simulink model "thermostat"  (R2014b)
settings: Solver=ode1  StartTime=0.0  StopTime=100  FixedStep=0.0001  MaxStep=0.0001  RelTol=1e-3
(part 1 of 2)
settings Model: Creator=sand080  LastModifiedBy=nall426
settings DataIOCC: LimitDataPoints=off
settings RTWCC: CustomInitializer=gettimeofday(&t0, 0);
settings RTWCC: CustomSourceCode=|
  | int gettimeofday(struct timeval * tp, struct timezone * tzp)
  | {
  |     // Note: some broken versions only have 8 trailing zero's, the correct epoch has 9 trailing zero's
  |     static const uint64_t EPOCH = ((uint64_t) 116444736000000000ULL);
  | 
  |     SYSTEMTIME  system_time;
  |     FILETIME    file_time;
  |     uint64_t    time;
  | 
  | 	GetSystemTime( &system_time );
  |     SystemTimeToFileTime( &system_time, &file_time );
  |     time =  ((uint64_t)file_time.dwLowDateTime )      ;
  |     time += ((uint64_t)file_time.dwHighDateTime) << 32;
  | 
  |     tp->tv_sec  = (long) ((time - EPOCH) / 10000000L);
  |     tp->tv_usec = (long) (system_time.wMilliseconds * 1000);
  |     return 0;
  | }
  | 
  | struct timeval t0, t1;
settings RTWCC: CustomHeaderCode=|
  | #include <stdint.h> // portable: uint64_t   MSVC: __int64
  | #include <Windows.h>
settings RTWCC: CustomTerminator=|
  | gettimeofday(&t1, 0);
  | 
  | long elapsed = (t1.tv_sec-t0.tv_sec)*1000000 + t1.tv_usec-t0.tv_usec;
  | printf("Time taken: %ld microseconds (%.3f seconds)\n", elapsed, (elapsed / 1000000.0));

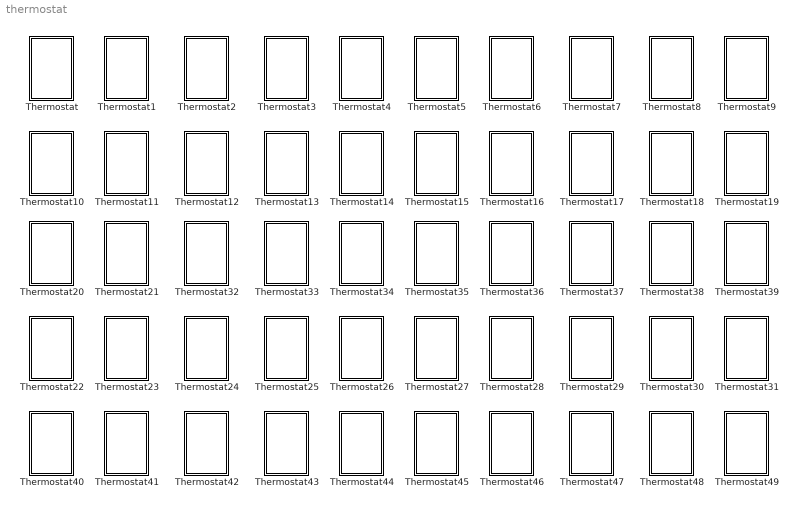
== system thermostat ==
  Thermostat : Subsystem
  Thermostat1 : Subsystem
  Thermostat10 : Subsystem
  Thermostat11 : Subsystem
  Thermostat12 : Subsystem
  Thermostat13 : Subsystem
  Thermostat14 : Subsystem
  Thermostat15 : Subsystem
  Thermostat16 : Subsystem
  Thermostat17 : Subsystem
  Thermostat18 : Subsystem
  Thermostat19 : Subsystem
  Thermostat2 : Subsystem
  Thermostat20 : Subsystem
  Thermostat21 : Subsystem
  Thermostat22 : Subsystem
  Thermostat23 : Subsystem
  Thermostat24 : Subsystem
  Thermostat25 : Subsystem
  Thermostat26 : Subsystem
  Thermostat27 : Subsystem
  Thermostat28 : Subsystem
  Thermostat29 : Subsystem
  Thermostat3 : Subsystem
  Thermostat30 : Subsystem
  Thermostat31 : Subsystem
  Thermostat32 : Subsystem
  Thermostat33 : Subsystem
  Thermostat34 : Subsystem
  Thermostat35 : Subsystem
  Thermostat36 : Subsystem
  Thermostat37 : Subsystem
  Thermostat38 : Subsystem
  Thermostat39 : Subsystem
  Thermostat4 : Subsystem
  Thermostat40 : Subsystem
  Thermostat41 : Subsystem
  Thermostat42 : Subsystem
  Thermostat43 : Subsystem
  Thermostat44 : Subsystem
  Thermostat45 : Subsystem
  Thermostat46 : Subsystem
  Thermostat47 : Subsystem
  Thermostat48 : Subsystem
  Thermostat49 : Subsystem
  Thermostat5 : Subsystem
  Thermostat6 : Subsystem
  Thermostat7 : Subsystem
  Thermostat8 : Subsystem
  Thermostat9 : Subsystem

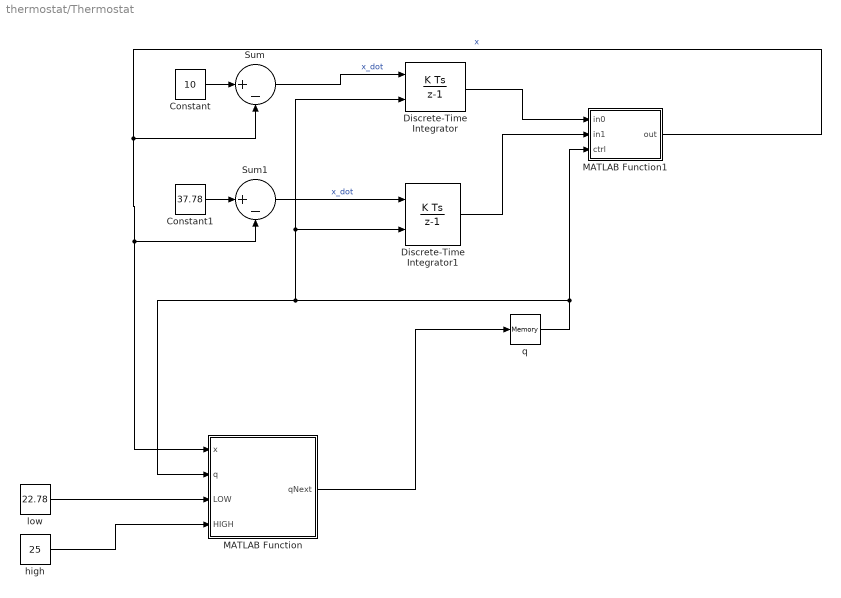
== system thermostat/Thermostat ==
  Constant : Constant  Value=10
  Constant1 : Constant  Value=37.78
  Discrete-Time Integrator : DiscreteIntegrator  ExternalReset=either  InitialCondition=25  InitialConditionSetting=State (most efficient)  SampleTime=-1
  Discrete-Time Integrator1 : DiscreteIntegrator  ExternalReset=either  InitialCondition=22.78  InitialConditionSetting=State (most efficient)  SampleTime=-1
  MATLAB Function : MATLAB Function  TreatAsAtomicUnit=on
  MATLAB Function1 : MATLAB Function  TreatAsAtomicUnit=on
  Sum : Sum  Inputs=|+-
  Sum1 : Sum  Inputs=|+-
  high : Constant  Value=25
  low : Constant  Value=22.78
  q : Memory
  wires:
  MATLAB Function/1(qNext) -> q/1
  Constant/1 -> Sum/1
  Sum/1 -> Discrete-Time Integrator/1  "x_dot"
  Discrete-Time Integrator1/1 -> MATLAB Function1/2(in1)
  Constant1/1 -> Sum1/1
  Sum1/1 -> Discrete-Time Integrator1/1  "x_dot"
  Discrete-Time Integrator/1 -> MATLAB Function1/1(in0)
  MATLAB Function1/1(out) -> Sum/2, MATLAB Function/1(x), Sum1/2  "x"
  low/1 -> MATLAB Function/3(LOW)
  high/1 -> MATLAB Function/4(HIGH)
  q/1 -> MATLAB Function1/3(ctrl), Discrete-Time Integrator1/2, Discrete-Time Integrator/2, MATLAB Function/2(q)

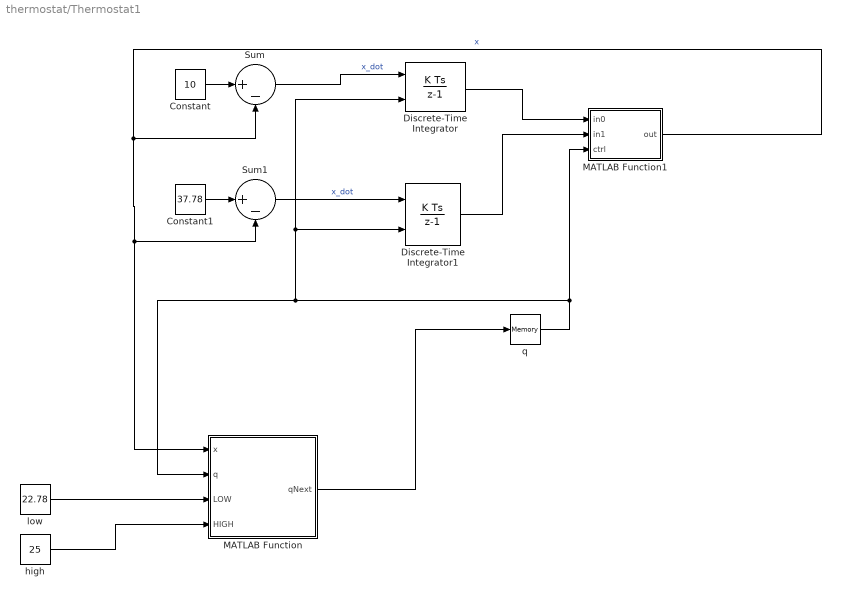
== system thermostat/Thermostat1 ==
  Constant : Constant  Value=10
  Constant1 : Constant  Value=37.78
  Discrete-Time Integrator : DiscreteIntegrator  ExternalReset=either  InitialCondition=25  InitialConditionSetting=State (most efficient)  SampleTime=-1
  Discrete-Time Integrator1 : DiscreteIntegrator  ExternalReset=either  InitialCondition=22.78  InitialConditionSetting=State (most efficient)  SampleTime=-1
  MATLAB Function : MATLAB Function  TreatAsAtomicUnit=on
  MATLAB Function1 : MATLAB Function  TreatAsAtomicUnit=on
  Sum : Sum  Inputs=|+-
  Sum1 : Sum  Inputs=|+-
  high : Constant  Value=25
  low : Constant  Value=22.78
  q : Memory
  wires:
  MATLAB Function/1(qNext) -> q/1
  Constant/1 -> Sum/1
  Sum/1 -> Discrete-Time Integrator/1  "x_dot"
  Discrete-Time Integrator1/1 -> MATLAB Function1/2(in1)
  Constant1/1 -> Sum1/1
  Sum1/1 -> Discrete-Time Integrator1/1  "x_dot"
  Discrete-Time Integrator/1 -> MATLAB Function1/1(in0)
  MATLAB Function1/1(out) -> Sum/2, MATLAB Function/1(x), Sum1/2  "x"
  low/1 -> MATLAB Function/3(LOW)
  high/1 -> MATLAB Function/4(HIGH)
  q/1 -> MATLAB Function1/3(ctrl), Discrete-Time Integrator1/2, Discrete-Time Integrator/2, MATLAB Function/2(q)

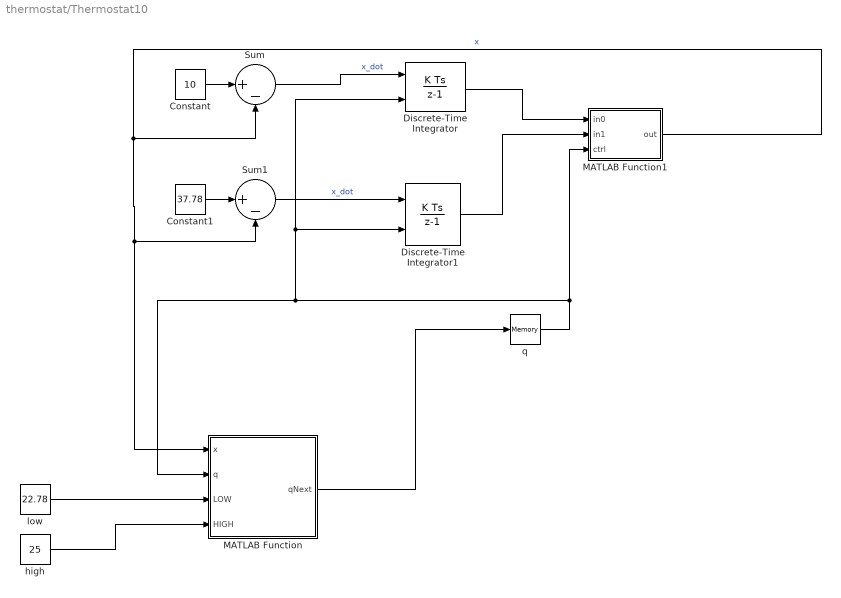
== system thermostat/Thermostat10 ==
  Constant : Constant  Value=10
  Constant1 : Constant  Value=37.78
  Discrete-Time Integrator : DiscreteIntegrator  ExternalReset=either  InitialCondition=25  InitialConditionSetting=State (most efficient)  SampleTime=-1
  Discrete-Time Integrator1 : DiscreteIntegrator  ExternalReset=either  InitialCondition=22.78  InitialConditionSetting=State (most efficient)  SampleTime=-1
  MATLAB Function : MATLAB Function  TreatAsAtomicUnit=on
  MATLAB Function1 : MATLAB Function  TreatAsAtomicUnit=on
  Sum : Sum  Inputs=|+-
  Sum1 : Sum  Inputs=|+-
  high : Constant  Value=25
  low : Constant  Value=22.78
  q : Memory
  wires:
  MATLAB Function/1(qNext) -> q/1
  Constant/1 -> Sum/1
  Sum/1 -> Discrete-Time Integrator/1  "x_dot"
  Discrete-Time Integrator1/1 -> MATLAB Function1/2(in1)
  Constant1/1 -> Sum1/1
  Sum1/1 -> Discrete-Time Integrator1/1  "x_dot"
  Discrete-Time Integrator/1 -> MATLAB Function1/1(in0)
  MATLAB Function1/1(out) -> Sum/2, MATLAB Function/1(x), Sum1/2  "x"
  low/1 -> MATLAB Function/3(LOW)
  high/1 -> MATLAB Function/4(HIGH)
  q/1 -> MATLAB Function1/3(ctrl), Discrete-Time Integrator1/2, Discrete-Time Integrator/2, MATLAB Function/2(q)

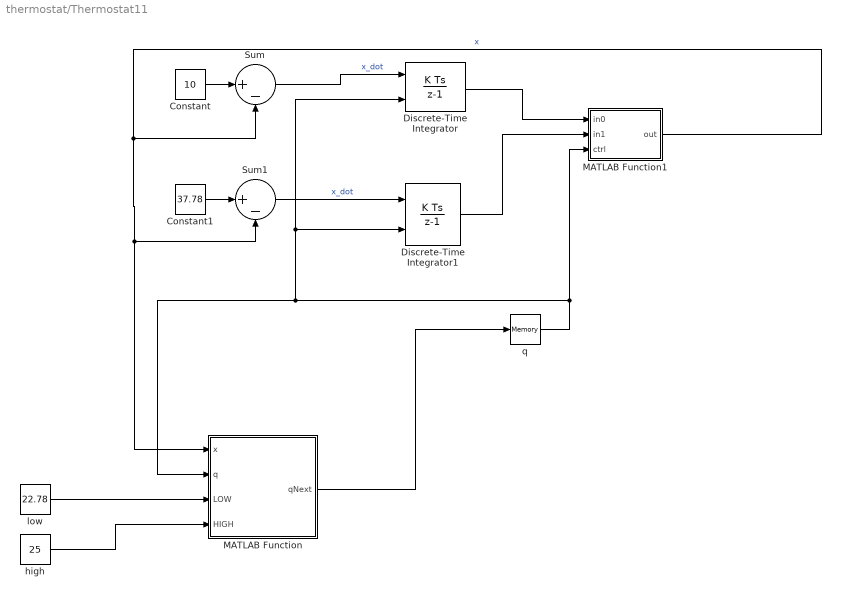
== system thermostat/Thermostat11 ==
  Constant : Constant  Value=10
  Constant1 : Constant  Value=37.78
  Discrete-Time Integrator : DiscreteIntegrator  ExternalReset=either  InitialCondition=25  InitialConditionSetting=State (most efficient)  SampleTime=-1
  Discrete-Time Integrator1 : DiscreteIntegrator  ExternalReset=either  InitialCondition=22.78  InitialConditionSetting=State (most efficient)  SampleTime=-1
  MATLAB Function : MATLAB Function  TreatAsAtomicUnit=on
  MATLAB Function1 : MATLAB Function  TreatAsAtomicUnit=on
  Sum : Sum  Inputs=|+-
  Sum1 : Sum  Inputs=|+-
  high : Constant  Value=25
  low : Constant  Value=22.78
  q : Memory
  wires:
  MATLAB Function/1(qNext) -> q/1
  Constant/1 -> Sum/1
  Sum/1 -> Discrete-Time Integrator/1  "x_dot"
  Discrete-Time Integrator1/1 -> MATLAB Function1/2(in1)
  Constant1/1 -> Sum1/1
  Sum1/1 -> Discrete-Time Integrator1/1  "x_dot"
  Discrete-Time Integrator/1 -> MATLAB Function1/1(in0)
  MATLAB Function1/1(out) -> Sum/2, MATLAB Function/1(x), Sum1/2  "x"
  low/1 -> MATLAB Function/3(LOW)
  high/1 -> MATLAB Function/4(HIGH)
  q/1 -> MATLAB Function1/3(ctrl), Discrete-Time Integrator1/2, Discrete-Time Integrator/2, MATLAB Function/2(q)

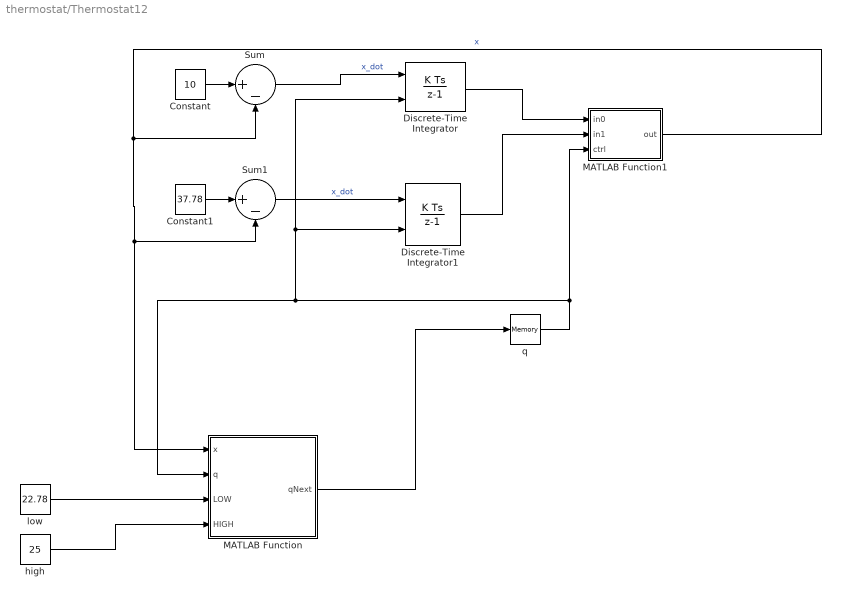
== system thermostat/Thermostat12 ==
  Constant : Constant  Value=10
  Constant1 : Constant  Value=37.78
  Discrete-Time Integrator : DiscreteIntegrator  ExternalReset=either  InitialCondition=25  InitialConditionSetting=State (most efficient)  SampleTime=-1
  Discrete-Time Integrator1 : DiscreteIntegrator  ExternalReset=either  InitialCondition=22.78  InitialConditionSetting=State (most efficient)  SampleTime=-1
  MATLAB Function : MATLAB Function  TreatAsAtomicUnit=on
  MATLAB Function1 : MATLAB Function  TreatAsAtomicUnit=on
  Sum : Sum  Inputs=|+-
  Sum1 : Sum  Inputs=|+-
  high : Constant  Value=25
  low : Constant  Value=22.78
  q : Memory
  wires:
  MATLAB Function/1(qNext) -> q/1
  Constant/1 -> Sum/1
  Sum/1 -> Discrete-Time Integrator/1  "x_dot"
  Discrete-Time Integrator1/1 -> MATLAB Function1/2(in1)
  Constant1/1 -> Sum1/1
  Sum1/1 -> Discrete-Time Integrator1/1  "x_dot"
  Discrete-Time Integrator/1 -> MATLAB Function1/1(in0)
  MATLAB Function1/1(out) -> Sum/2, MATLAB Function/1(x), Sum1/2  "x"
  low/1 -> MATLAB Function/3(LOW)
  high/1 -> MATLAB Function/4(HIGH)
  q/1 -> MATLAB Function1/3(ctrl), Discrete-Time Integrator1/2, Discrete-Time Integrator/2, MATLAB Function/2(q)

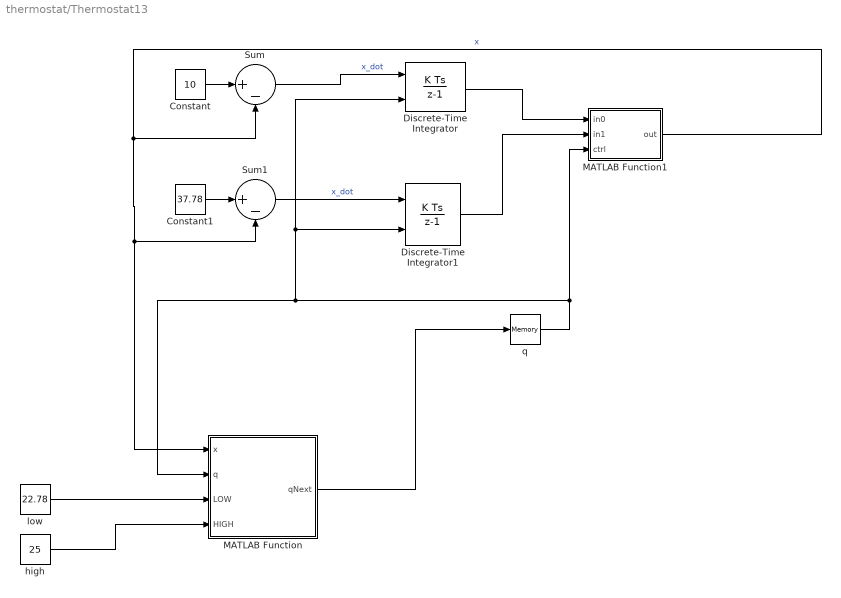
== system thermostat/Thermostat13 ==
  Constant : Constant  Value=10
  Constant1 : Constant  Value=37.78
  Discrete-Time Integrator : DiscreteIntegrator  ExternalReset=either  InitialCondition=25  InitialConditionSetting=State (most efficient)  SampleTime=-1
  Discrete-Time Integrator1 : DiscreteIntegrator  ExternalReset=either  InitialCondition=22.78  InitialConditionSetting=State (most efficient)  SampleTime=-1
  MATLAB Function : MATLAB Function  TreatAsAtomicUnit=on
  MATLAB Function1 : MATLAB Function  TreatAsAtomicUnit=on
  Sum : Sum  Inputs=|+-
  Sum1 : Sum  Inputs=|+-
  high : Constant  Value=25
  low : Constant  Value=22.78
  q : Memory
  wires:
  MATLAB Function/1(qNext) -> q/1
  Constant/1 -> Sum/1
  Sum/1 -> Discrete-Time Integrator/1  "x_dot"
  Discrete-Time Integrator1/1 -> MATLAB Function1/2(in1)
  Constant1/1 -> Sum1/1
  Sum1/1 -> Discrete-Time Integrator1/1  "x_dot"
  Discrete-Time Integrator/1 -> MATLAB Function1/1(in0)
  MATLAB Function1/1(out) -> Sum/2, MATLAB Function/1(x), Sum1/2  "x"
  low/1 -> MATLAB Function/3(LOW)
  high/1 -> MATLAB Function/4(HIGH)
  q/1 -> MATLAB Function1/3(ctrl), Discrete-Time Integrator1/2, Discrete-Time Integrator/2, MATLAB Function/2(q)

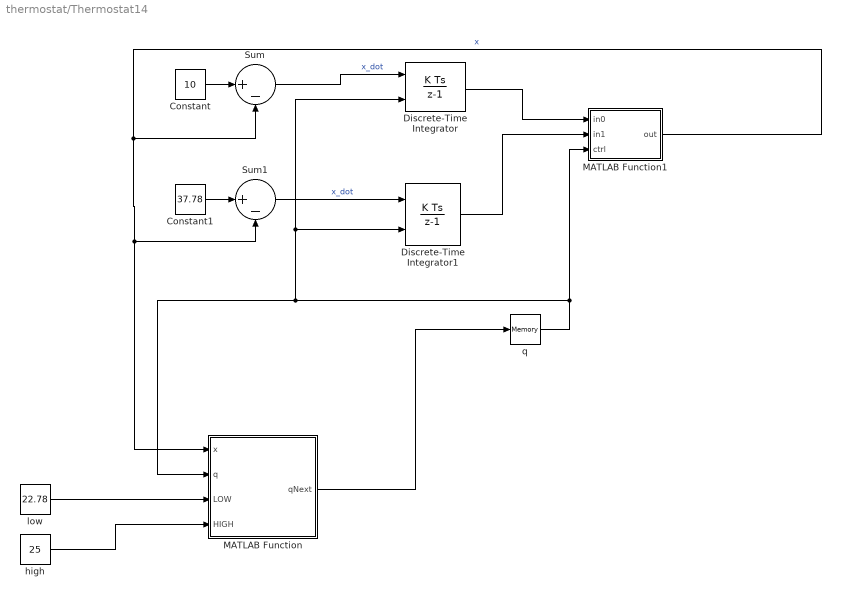
== system thermostat/Thermostat14 ==
  Constant : Constant  Value=10
  Constant1 : Constant  Value=37.78
  Discrete-Time Integrator : DiscreteIntegrator  ExternalReset=either  InitialCondition=25  InitialConditionSetting=State (most efficient)  SampleTime=-1
  Discrete-Time Integrator1 : DiscreteIntegrator  ExternalReset=either  InitialCondition=22.78  InitialConditionSetting=State (most efficient)  SampleTime=-1
  MATLAB Function : MATLAB Function  TreatAsAtomicUnit=on
  MATLAB Function1 : MATLAB Function  TreatAsAtomicUnit=on
  Sum : Sum  Inputs=|+-
  Sum1 : Sum  Inputs=|+-
  high : Constant  Value=25
  low : Constant  Value=22.78
  q : Memory
  wires:
  MATLAB Function/1(qNext) -> q/1
  Constant/1 -> Sum/1
  Sum/1 -> Discrete-Time Integrator/1  "x_dot"
  Discrete-Time Integrator1/1 -> MATLAB Function1/2(in1)
  Constant1/1 -> Sum1/1
  Sum1/1 -> Discrete-Time Integrator1/1  "x_dot"
  Discrete-Time Integrator/1 -> MATLAB Function1/1(in0)
  MATLAB Function1/1(out) -> Sum/2, MATLAB Function/1(x), Sum1/2  "x"
  low/1 -> MATLAB Function/3(LOW)
  high/1 -> MATLAB Function/4(HIGH)
  q/1 -> MATLAB Function1/3(ctrl), Discrete-Time Integrator1/2, Discrete-Time Integrator/2, MATLAB Function/2(q)

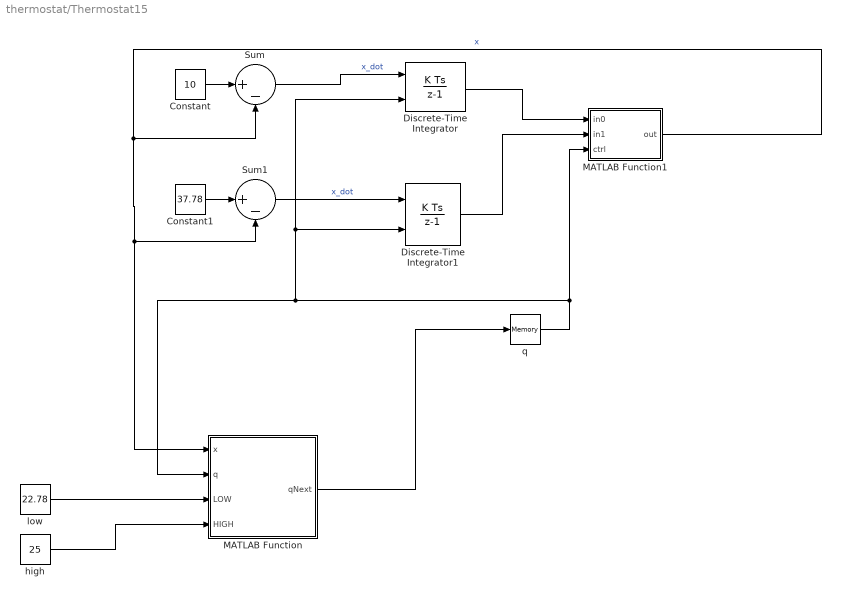
== system thermostat/Thermostat15 ==
  Constant : Constant  Value=10
  Constant1 : Constant  Value=37.78
  Discrete-Time Integrator : DiscreteIntegrator  ExternalReset=either  InitialCondition=25  InitialConditionSetting=State (most efficient)  SampleTime=-1
  Discrete-Time Integrator1 : DiscreteIntegrator  ExternalReset=either  InitialCondition=22.78  InitialConditionSetting=State (most efficient)  SampleTime=-1
  MATLAB Function : MATLAB Function  TreatAsAtomicUnit=on
  MATLAB Function1 : MATLAB Function  TreatAsAtomicUnit=on
  Sum : Sum  Inputs=|+-
  Sum1 : Sum  Inputs=|+-
  high : Constant  Value=25
  low : Constant  Value=22.78
  q : Memory
  wires:
  MATLAB Function/1(qNext) -> q/1
  Constant/1 -> Sum/1
  Sum/1 -> Discrete-Time Integrator/1  "x_dot"
  Discrete-Time Integrator1/1 -> MATLAB Function1/2(in1)
  Constant1/1 -> Sum1/1
  Sum1/1 -> Discrete-Time Integrator1/1  "x_dot"
  Discrete-Time Integrator/1 -> MATLAB Function1/1(in0)
  MATLAB Function1/1(out) -> Sum/2, MATLAB Function/1(x), Sum1/2  "x"
  low/1 -> MATLAB Function/3(LOW)
  high/1 -> MATLAB Function/4(HIGH)
  q/1 -> MATLAB Function1/3(ctrl), Discrete-Time Integrator1/2, Discrete-Time Integrator/2, MATLAB Function/2(q)

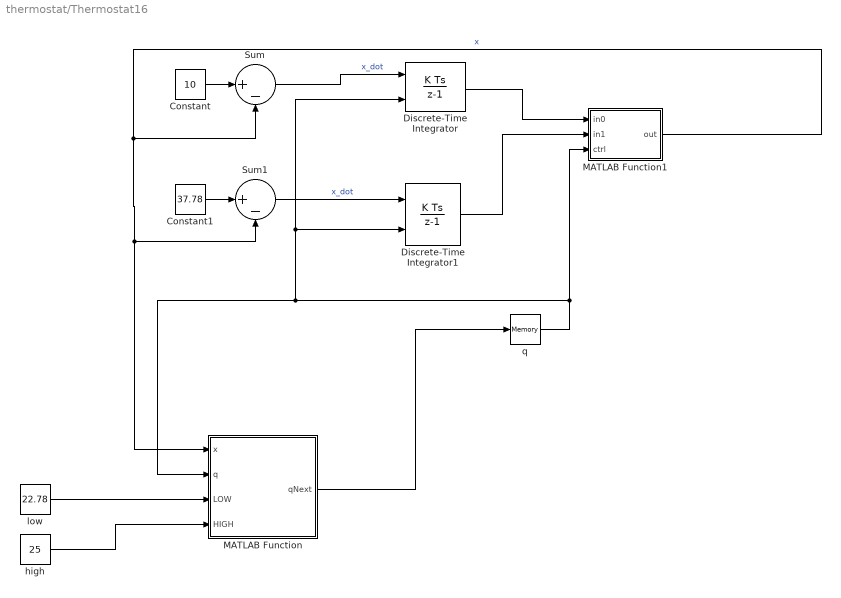
== system thermostat/Thermostat16 ==
  Constant : Constant  Value=10
  Constant1 : Constant  Value=37.78
  Discrete-Time Integrator : DiscreteIntegrator  ExternalReset=either  InitialCondition=25  InitialConditionSetting=State (most efficient)  SampleTime=-1
  Discrete-Time Integrator1 : DiscreteIntegrator  ExternalReset=either  InitialCondition=22.78  InitialConditionSetting=State (most efficient)  SampleTime=-1
  MATLAB Function : MATLAB Function  TreatAsAtomicUnit=on
  MATLAB Function1 : MATLAB Function  TreatAsAtomicUnit=on
  Sum : Sum  Inputs=|+-
  Sum1 : Sum  Inputs=|+-
  high : Constant  Value=25
  low : Constant  Value=22.78
  q : Memory
  wires:
  MATLAB Function/1(qNext) -> q/1
  Constant/1 -> Sum/1
  Sum/1 -> Discrete-Time Integrator/1  "x_dot"
  Discrete-Time Integrator1/1 -> MATLAB Function1/2(in1)
  Constant1/1 -> Sum1/1
  Sum1/1 -> Discrete-Time Integrator1/1  "x_dot"
  Discrete-Time Integrator/1 -> MATLAB Function1/1(in0)
  MATLAB Function1/1(out) -> Sum/2, MATLAB Function/1(x), Sum1/2  "x"
  low/1 -> MATLAB Function/3(LOW)
  high/1 -> MATLAB Function/4(HIGH)
  q/1 -> MATLAB Function1/3(ctrl), Discrete-Time Integrator1/2, Discrete-Time Integrator/2, MATLAB Function/2(q)

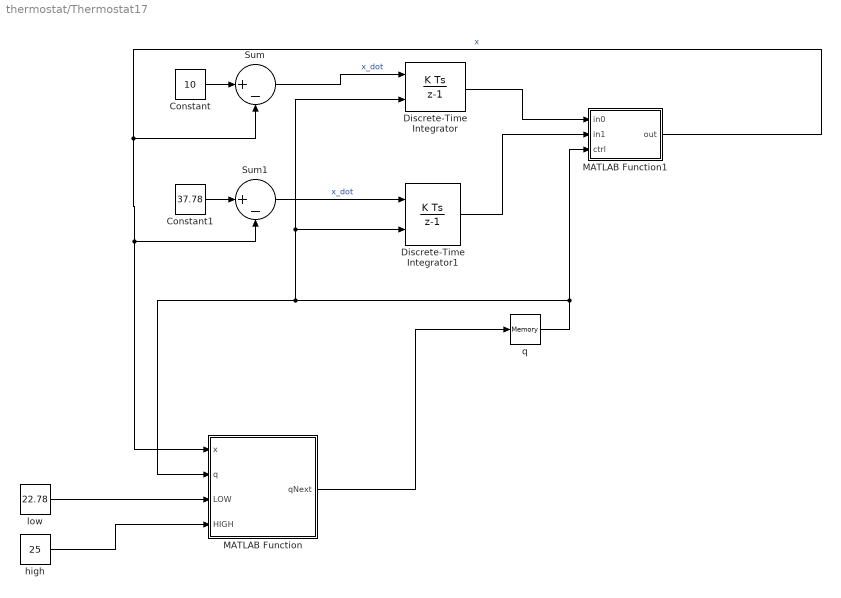
== system thermostat/Thermostat17 ==
  Constant : Constant  Value=10
  Constant1 : Constant  Value=37.78
  Discrete-Time Integrator : DiscreteIntegrator  ExternalReset=either  InitialCondition=25  InitialConditionSetting=State (most efficient)  SampleTime=-1
  Discrete-Time Integrator1 : DiscreteIntegrator  ExternalReset=either  InitialCondition=22.78  InitialConditionSetting=State (most efficient)  SampleTime=-1
  MATLAB Function : MATLAB Function  TreatAsAtomicUnit=on
  MATLAB Function1 : MATLAB Function  TreatAsAtomicUnit=on
  Sum : Sum  Inputs=|+-
  Sum1 : Sum  Inputs=|+-
  high : Constant  Value=25
  low : Constant  Value=22.78
  q : Memory
  wires:
  MATLAB Function/1(qNext) -> q/1
  Constant/1 -> Sum/1
  Sum/1 -> Discrete-Time Integrator/1  "x_dot"
  Discrete-Time Integrator1/1 -> MATLAB Function1/2(in1)
  Constant1/1 -> Sum1/1
  Sum1/1 -> Discrete-Time Integrator1/1  "x_dot"
  Discrete-Time Integrator/1 -> MATLAB Function1/1(in0)
  MATLAB Function1/1(out) -> Sum/2, MATLAB Function/1(x), Sum1/2  "x"
  low/1 -> MATLAB Function/3(LOW)
  high/1 -> MATLAB Function/4(HIGH)
  q/1 -> MATLAB Function1/3(ctrl), Discrete-Time Integrator1/2, Discrete-Time Integrator/2, MATLAB Function/2(q)

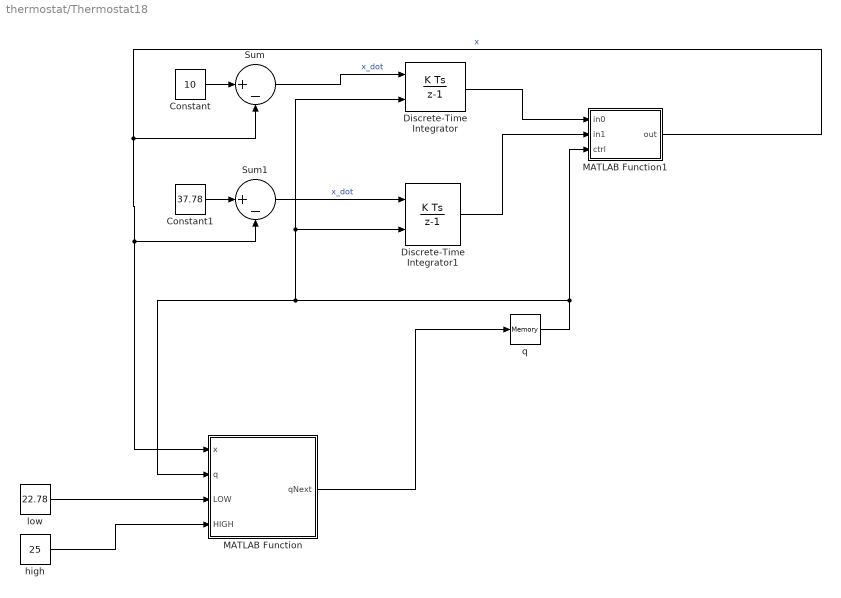
== system thermostat/Thermostat18 ==
  Constant : Constant  Value=10
  Constant1 : Constant  Value=37.78
  Discrete-Time Integrator : DiscreteIntegrator  ExternalReset=either  InitialCondition=25  InitialConditionSetting=State (most efficient)  SampleTime=-1
  Discrete-Time Integrator1 : DiscreteIntegrator  ExternalReset=either  InitialCondition=22.78  InitialConditionSetting=State (most efficient)  SampleTime=-1
  MATLAB Function : MATLAB Function  TreatAsAtomicUnit=on
  MATLAB Function1 : MATLAB Function  TreatAsAtomicUnit=on
  Sum : Sum  Inputs=|+-
  Sum1 : Sum  Inputs=|+-
  high : Constant  Value=25
  low : Constant  Value=22.78
  q : Memory
  wires:
  MATLAB Function/1(qNext) -> q/1
  Constant/1 -> Sum/1
  Sum/1 -> Discrete-Time Integrator/1  "x_dot"
  Discrete-Time Integrator1/1 -> MATLAB Function1/2(in1)
  Constant1/1 -> Sum1/1
  Sum1/1 -> Discrete-Time Integrator1/1  "x_dot"
  Discrete-Time Integrator/1 -> MATLAB Function1/1(in0)
  MATLAB Function1/1(out) -> Sum/2, MATLAB Function/1(x), Sum1/2  "x"
  low/1 -> MATLAB Function/3(LOW)
  high/1 -> MATLAB Function/4(HIGH)
  q/1 -> MATLAB Function1/3(ctrl), Discrete-Time Integrator1/2, Discrete-Time Integrator/2, MATLAB Function/2(q)

== system thermostat/Thermostat19 ==
  Constant : Constant  Value=10
  Constant1 : Constant  Value=37.78
  Discrete-Time Integrator : DiscreteIntegrator  ExternalReset=either  InitialCondition=25  InitialConditionSetting=State (most efficient)  SampleTime=-1
  Discrete-Time Integrator1 : DiscreteIntegrator  ExternalReset=either  InitialCondition=22.78  InitialConditionSetting=State (most efficient)  SampleTime=-1
  MATLAB Function : MATLAB Function  TreatAsAtomicUnit=on
  MATLAB Function1 : MATLAB Function  TreatAsAtomicUnit=on
  Sum : Sum  Inputs=|+-
  Sum1 : Sum  Inputs=|+-
  high : Constant  Value=25
  low : Constant  Value=22.78
  q : Memory
  wires:
  MATLAB Function/1(qNext) -> q/1
  Constant/1 -> Sum/1
  Sum/1 -> Discrete-Time Integrator/1  "x_dot"
  Discrete-Time Integrator1/1 -> MATLAB Function1/2(in1)
  Constant1/1 -> Sum1/1
  Sum1/1 -> Discrete-Time Integrator1/1  "x_dot"
  Discrete-Time Integrator/1 -> MATLAB Function1/1(in0)
  MATLAB Function1/1(out) -> Sum/2, MATLAB Function/1(x), Sum1/2  "x"
  low/1 -> MATLAB Function/3(LOW)
  high/1 -> MATLAB Function/4(HIGH)
  q/1 -> MATLAB Function1/3(ctrl), Discrete-Time Integrator1/2, Discrete-Time Integrator/2, MATLAB Function/2(q)

== system thermostat/Thermostat2 ==
  Constant : Constant  Value=10
  Constant1 : Constant  Value=37.78
  Discrete-Time Integrator : DiscreteIntegrator  ExternalReset=either  InitialCondition=25  InitialConditionSetting=State (most efficient)  SampleTime=-1
  Discrete-Time Integrator1 : DiscreteIntegrator  ExternalReset=either  InitialCondition=22.78  InitialConditionSetting=State (most efficient)  SampleTime=-1
  MATLAB Function : MATLAB Function  TreatAsAtomicUnit=on
  MATLAB Function1 : MATLAB Function  TreatAsAtomicUnit=on
  Sum : Sum  Inputs=|+-
  Sum1 : Sum  Inputs=|+-
  high : Constant  Value=25
  low : Constant  Value=22.78
  q : Memory
  wires:
  MATLAB Function/1(qNext) -> q/1
  Constant/1 -> Sum/1
  Sum/1 -> Discrete-Time Integrator/1  "x_dot"
  Discrete-Time Integrator1/1 -> MATLAB Function1/2(in1)
  Constant1/1 -> Sum1/1
  Sum1/1 -> Discrete-Time Integrator1/1  "x_dot"
  Discrete-Time Integrator/1 -> MATLAB Function1/1(in0)
  MATLAB Function1/1(out) -> Sum/2, MATLAB Function/1(x), Sum1/2  "x"
  low/1 -> MATLAB Function/3(LOW)
  high/1 -> MATLAB Function/4(HIGH)
  q/1 -> MATLAB Function1/3(ctrl), Discrete-Time Integrator1/2, Discrete-Time Integrator/2, MATLAB Function/2(q)

== system thermostat/Thermostat20 ==
  Constant : Constant  Value=10
  Constant1 : Constant  Value=37.78
  Discrete-Time Integrator : DiscreteIntegrator  ExternalReset=either  InitialCondition=25  InitialConditionSetting=State (most efficient)  SampleTime=-1
  Discrete-Time Integrator1 : DiscreteIntegrator  ExternalReset=either  InitialCondition=22.78  InitialConditionSetting=State (most efficient)  SampleTime=-1
  MATLAB Function : MATLAB Function  TreatAsAtomicUnit=on
  MATLAB Function1 : MATLAB Function  TreatAsAtomicUnit=on
  Sum : Sum  Inputs=|+-
  Sum1 : Sum  Inputs=|+-
  high : Constant  Value=25
  low : Constant  Value=22.78
  q : Memory
  wires:
  MATLAB Function/1(qNext) -> q/1
  Constant/1 -> Sum/1
  Sum/1 -> Discrete-Time Integrator/1  "x_dot"
  Discrete-Time Integrator1/1 -> MATLAB Function1/2(in1)
  Constant1/1 -> Sum1/1
  Sum1/1 -> Discrete-Time Integrator1/1  "x_dot"
  Discrete-Time Integrator/1 -> MATLAB Function1/1(in0)
  MATLAB Function1/1(out) -> Sum/2, MATLAB Function/1(x), Sum1/2  "x"
  low/1 -> MATLAB Function/3(LOW)
  high/1 -> MATLAB Function/4(HIGH)
  q/1 -> MATLAB Function1/3(ctrl), Discrete-Time Integrator1/2, Discrete-Time Integrator/2, MATLAB Function/2(q)

== system thermostat/Thermostat21 ==
  Constant : Constant  Value=10
  Constant1 : Constant  Value=37.78
  Discrete-Time Integrator : DiscreteIntegrator  ExternalReset=either  InitialCondition=25  InitialConditionSetting=State (most efficient)  SampleTime=-1
  Discrete-Time Integrator1 : DiscreteIntegrator  ExternalReset=either  InitialCondition=22.78  InitialConditionSetting=State (most efficient)  SampleTime=-1
  MATLAB Function : MATLAB Function  TreatAsAtomicUnit=on
  MATLAB Function1 : MATLAB Function  TreatAsAtomicUnit=on
  Sum : Sum  Inputs=|+-
  Sum1 : Sum  Inputs=|+-
  high : Constant  Value=25
  low : Constant  Value=22.78
  q : Memory
  wires:
  MATLAB Function/1(qNext) -> q/1
  Constant/1 -> Sum/1
  Sum/1 -> Discrete-Time Integrator/1  "x_dot"
  Discrete-Time Integrator1/1 -> MATLAB Function1/2(in1)
  Constant1/1 -> Sum1/1
  Sum1/1 -> Discrete-Time Integrator1/1  "x_dot"
  Discrete-Time Integrator/1 -> MATLAB Function1/1(in0)
  MATLAB Function1/1(out) -> Sum/2, MATLAB Function/1(x), Sum1/2  "x"
  low/1 -> MATLAB Function/3(LOW)
  high/1 -> MATLAB Function/4(HIGH)
  q/1 -> MATLAB Function1/3(ctrl), Discrete-Time Integrator1/2, Discrete-Time Integrator/2, MATLAB Function/2(q)

== system thermostat/Thermostat22 ==
  Constant : Constant  Value=10
  Constant1 : Constant  Value=37.78
  Discrete-Time Integrator : DiscreteIntegrator  ExternalReset=either  InitialCondition=25  InitialConditionSetting=State (most efficient)  SampleTime=-1
  Discrete-Time Integrator1 : DiscreteIntegrator  ExternalReset=either  InitialCondition=22.78  InitialConditionSetting=State (most efficient)  SampleTime=-1
  MATLAB Function : MATLAB Function  TreatAsAtomicUnit=on
  MATLAB Function1 : MATLAB Function  TreatAsAtomicUnit=on
  Sum : Sum  Inputs=|+-
  Sum1 : Sum  Inputs=|+-
  high : Constant  Value=25
  low : Constant  Value=22.78
  q : Memory
  wires:
  MATLAB Function/1(qNext) -> q/1
  Constant/1 -> Sum/1
  Sum/1 -> Discrete-Time Integrator/1  "x_dot"
  Discrete-Time Integrator1/1 -> MATLAB Function1/2(in1)
  Constant1/1 -> Sum1/1
  Sum1/1 -> Discrete-Time Integrator1/1  "x_dot"
  Discrete-Time Integrator/1 -> MATLAB Function1/1(in0)
  MATLAB Function1/1(out) -> Sum/2, MATLAB Function/1(x), Sum1/2  "x"
  low/1 -> MATLAB Function/3(LOW)
  high/1 -> MATLAB Function/4(HIGH)
  q/1 -> MATLAB Function1/3(ctrl), Discrete-Time Integrator1/2, Discrete-Time Integrator/2, MATLAB Function/2(q)

== system thermostat/Thermostat23 ==
  Constant : Constant  Value=10
  Constant1 : Constant  Value=37.78
  Discrete-Time Integrator : DiscreteIntegrator  ExternalReset=either  InitialCondition=25  InitialConditionSetting=State (most efficient)  SampleTime=-1
  Discrete-Time Integrator1 : DiscreteIntegrator  ExternalReset=either  InitialCondition=22.78  InitialConditionSetting=State (most efficient)  SampleTime=-1
  MATLAB Function : MATLAB Function  TreatAsAtomicUnit=on
  MATLAB Function1 : MATLAB Function  TreatAsAtomicUnit=on
  Sum : Sum  Inputs=|+-
  Sum1 : Sum  Inputs=|+-
  high : Constant  Value=25
  low : Constant  Value=22.78
  q : Memory
  wires:
  MATLAB Function/1(qNext) -> q/1
  Constant/1 -> Sum/1
  Sum/1 -> Discrete-Time Integrator/1  "x_dot"
  Discrete-Time Integrator1/1 -> MATLAB Function1/2(in1)
  Constant1/1 -> Sum1/1
  Sum1/1 -> Discrete-Time Integrator1/1  "x_dot"
  Discrete-Time Integrator/1 -> MATLAB Function1/1(in0)
  MATLAB Function1/1(out) -> Sum/2, MATLAB Function/1(x), Sum1/2  "x"
  low/1 -> MATLAB Function/3(LOW)
  high/1 -> MATLAB Function/4(HIGH)
  q/1 -> MATLAB Function1/3(ctrl), Discrete-Time Integrator1/2, Discrete-Time Integrator/2, MATLAB Function/2(q)

== system thermostat/Thermostat24 ==
  Constant : Constant  Value=10
  Constant1 : Constant  Value=37.78
  Discrete-Time Integrator : DiscreteIntegrator  ExternalReset=either  InitialCondition=25  InitialConditionSetting=State (most efficient)  SampleTime=-1
  Discrete-Time Integrator1 : DiscreteIntegrator  ExternalReset=either  InitialCondition=22.78  InitialConditionSetting=State (most efficient)  SampleTime=-1
  MATLAB Function : MATLAB Function  TreatAsAtomicUnit=on
  MATLAB Function1 : MATLAB Function  TreatAsAtomicUnit=on
  Sum : Sum  Inputs=|+-
  Sum1 : Sum  Inputs=|+-
  high : Constant  Value=25
  low : Constant  Value=22.78
  q : Memory
  wires:
  MATLAB Function/1(qNext) -> q/1
  Constant/1 -> Sum/1
  Sum/1 -> Discrete-Time Integrator/1  "x_dot"
  Discrete-Time Integrator1/1 -> MATLAB Function1/2(in1)
  Constant1/1 -> Sum1/1
  Sum1/1 -> Discrete-Time Integrator1/1  "x_dot"
  Discrete-Time Integrator/1 -> MATLAB Function1/1(in0)
  MATLAB Function1/1(out) -> Sum/2, MATLAB Function/1(x), Sum1/2  "x"
  low/1 -> MATLAB Function/3(LOW)
  high/1 -> MATLAB Function/4(HIGH)
  q/1 -> MATLAB Function1/3(ctrl), Discrete-Time Integrator1/2, Discrete-Time Integrator/2, MATLAB Function/2(q)

== system thermostat/Thermostat25 ==
  Constant : Constant  Value=10
  Constant1 : Constant  Value=37.78
  Discrete-Time Integrator : DiscreteIntegrator  ExternalReset=either  InitialCondition=25  InitialConditionSetting=State (most efficient)  SampleTime=-1
  Discrete-Time Integrator1 : DiscreteIntegrator  ExternalReset=either  InitialCondition=22.78  InitialConditionSetting=State (most efficient)  SampleTime=-1
  MATLAB Function : MATLAB Function  TreatAsAtomicUnit=on
  MATLAB Function1 : MATLAB Function  TreatAsAtomicUnit=on
  Sum : Sum  Inputs=|+-
  Sum1 : Sum  Inputs=|+-
  high : Constant  Value=25
  low : Constant  Value=22.78
  q : Memory
  wires:
  MATLAB Function/1(qNext) -> q/1
  Constant/1 -> Sum/1
  Sum/1 -> Discrete-Time Integrator/1  "x_dot"
  Discrete-Time Integrator1/1 -> MATLAB Function1/2(in1)
  Constant1/1 -> Sum1/1
  Sum1/1 -> Discrete-Time Integrator1/1  "x_dot"
  Discrete-Time Integrator/1 -> MATLAB Function1/1(in0)
  MATLAB Function1/1(out) -> Sum/2, MATLAB Function/1(x), Sum1/2  "x"
  low/1 -> MATLAB Function/3(LOW)
  high/1 -> MATLAB Function/4(HIGH)
  q/1 -> MATLAB Function1/3(ctrl), Discrete-Time Integrator1/2, Discrete-Time Integrator/2, MATLAB Function/2(q)

== system thermostat/Thermostat26 ==
  Constant : Constant  Value=10
  Constant1 : Constant  Value=37.78
  Discrete-Time Integrator : DiscreteIntegrator  ExternalReset=either  InitialCondition=25  InitialConditionSetting=State (most efficient)  SampleTime=-1
  Discrete-Time Integrator1 : DiscreteIntegrator  ExternalReset=either  InitialCondition=22.78  InitialConditionSetting=State (most efficient)  SampleTime=-1
  MATLAB Function : MATLAB Function  TreatAsAtomicUnit=on
  MATLAB Function1 : MATLAB Function  TreatAsAtomicUnit=on
  Sum : Sum  Inputs=|+-
  Sum1 : Sum  Inputs=|+-
  high : Constant  Value=25
  low : Constant  Value=22.78
  q : Memory
  wires:
  MATLAB Function/1(qNext) -> q/1
  Constant/1 -> Sum/1
  Sum/1 -> Discrete-Time Integrator/1  "x_dot"
  Discrete-Time Integrator1/1 -> MATLAB Function1/2(in1)
  Constant1/1 -> Sum1/1
  Sum1/1 -> Discrete-Time Integrator1/1  "x_dot"
  Discrete-Time Integrator/1 -> MATLAB Function1/1(in0)
  MATLAB Function1/1(out) -> Sum/2, MATLAB Function/1(x), Sum1/2  "x"
  low/1 -> MATLAB Function/3(LOW)
  high/1 -> MATLAB Function/4(HIGH)
  q/1 -> MATLAB Function1/3(ctrl), Discrete-Time Integrator1/2, Discrete-Time Integrator/2, MATLAB Function/2(q)

== system thermostat/Thermostat27 ==
  Constant : Constant  Value=10
  Constant1 : Constant  Value=37.78
  Discrete-Time Integrator : DiscreteIntegrator  ExternalReset=either  InitialCondition=25  InitialConditionSetting=State (most efficient)  SampleTime=-1
  Discrete-Time Integrator1 : DiscreteIntegrator  ExternalReset=either  InitialCondition=22.78  InitialConditionSetting=State (most efficient)  SampleTime=-1
  MATLAB Function : MATLAB Function  TreatAsAtomicUnit=on
  MATLAB Function1 : MATLAB Function  TreatAsAtomicUnit=on
  Sum : Sum  Inputs=|+-
  Sum1 : Sum  Inputs=|+-
  high : Constant  Value=25
  low : Constant  Value=22.78
  q : Memory
  wires:
  MATLAB Function/1(qNext) -> q/1
  Constant/1 -> Sum/1
  Sum/1 -> Discrete-Time Integrator/1  "x_dot"
  Discrete-Time Integrator1/1 -> MATLAB Function1/2(in1)
  Constant1/1 -> Sum1/1
  Sum1/1 -> Discrete-Time Integrator1/1  "x_dot"
  Discrete-Time Integrator/1 -> MATLAB Function1/1(in0)
  MATLAB Function1/1(out) -> Sum/2, MATLAB Function/1(x), Sum1/2  "x"
  low/1 -> MATLAB Function/3(LOW)
  high/1 -> MATLAB Function/4(HIGH)
  q/1 -> MATLAB Function1/3(ctrl), Discrete-Time Integrator1/2, Discrete-Time Integrator/2, MATLAB Function/2(q)

== system thermostat/Thermostat28 ==
  Constant : Constant  Value=10
  Constant1 : Constant  Value=37.78
  Discrete-Time Integrator : DiscreteIntegrator  ExternalReset=either  InitialCondition=25  InitialConditionSetting=State (most efficient)  SampleTime=-1
  Discrete-Time Integrator1 : DiscreteIntegrator  ExternalReset=either  InitialCondition=22.78  InitialConditionSetting=State (most efficient)  SampleTime=-1
  MATLAB Function : MATLAB Function  TreatAsAtomicUnit=on
  MATLAB Function1 : MATLAB Function  TreatAsAtomicUnit=on
  Sum : Sum  Inputs=|+-
  Sum1 : Sum  Inputs=|+-
  high : Constant  Value=25
  low : Constant  Value=22.78
  q : Memory
  wires:
  MATLAB Function/1(qNext) -> q/1
  Constant/1 -> Sum/1
  Sum/1 -> Discrete-Time Integrator/1  "x_dot"
  Discrete-Time Integrator1/1 -> MATLAB Function1/2(in1)
  Constant1/1 -> Sum1/1
  Sum1/1 -> Discrete-Time Integrator1/1  "x_dot"
  Discrete-Time Integrator/1 -> MATLAB Function1/1(in0)
  MATLAB Function1/1(out) -> Sum/2, MATLAB Function/1(x), Sum1/2  "x"
  low/1 -> MATLAB Function/3(LOW)
  high/1 -> MATLAB Function/4(HIGH)
  q/1 -> MATLAB Function1/3(ctrl), Discrete-Time Integrator1/2, Discrete-Time Integrator/2, MATLAB Function/2(q)

== system thermostat/Thermostat29 ==
  Constant : Constant  Value=10
  Constant1 : Constant  Value=37.78
  Discrete-Time Integrator : DiscreteIntegrator  ExternalReset=either  InitialCondition=25  InitialConditionSetting=State (most efficient)  SampleTime=-1
  Discrete-Time Integrator1 : DiscreteIntegrator  ExternalReset=either  InitialCondition=22.78  InitialConditionSetting=State (most efficient)  SampleTime=-1
  MATLAB Function : MATLAB Function  TreatAsAtomicUnit=on
  MATLAB Function1 : MATLAB Function  TreatAsAtomicUnit=on
  Sum : Sum  Inputs=|+-
  Sum1 : Sum  Inputs=|+-
  high : Constant  Value=25
  low : Constant  Value=22.78
  q : Memory
  wires:
  MATLAB Function/1(qNext) -> q/1
  Constant/1 -> Sum/1
  Sum/1 -> Discrete-Time Integrator/1  "x_dot"
  Discrete-Time Integrator1/1 -> MATLAB Function1/2(in1)
  Constant1/1 -> Sum1/1
  Sum1/1 -> Discrete-Time Integrator1/1  "x_dot"
  Discrete-Time Integrator/1 -> MATLAB Function1/1(in0)
  MATLAB Function1/1(out) -> Sum/2, MATLAB Function/1(x), Sum1/2  "x"
  low/1 -> MATLAB Function/3(LOW)
  high/1 -> MATLAB Function/4(HIGH)
  q/1 -> MATLAB Function1/3(ctrl), Discrete-Time Integrator1/2, Discrete-Time Integrator/2, MATLAB Function/2(q)

== system thermostat/Thermostat3 ==
  Constant : Constant  Value=10
  Constant1 : Constant  Value=37.78
  Discrete-Time Integrator : DiscreteIntegrator  ExternalReset=either  InitialCondition=25  InitialConditionSetting=State (most efficient)  SampleTime=-1
  Discrete-Time Integrator1 : DiscreteIntegrator  ExternalReset=either  InitialCondition=22.78  InitialConditionSetting=State (most efficient)  SampleTime=-1
  MATLAB Function : MATLAB Function  TreatAsAtomicUnit=on
  MATLAB Function1 : MATLAB Function  TreatAsAtomicUnit=on
  Sum : Sum  Inputs=|+-
  Sum1 : Sum  Inputs=|+-
  high : Constant  Value=25
  low : Constant  Value=22.78
  q : Memory
  wires:
  MATLAB Function/1(qNext) -> q/1
  Constant/1 -> Sum/1
  Sum/1 -> Discrete-Time Integrator/1  "x_dot"
  Discrete-Time Integrator1/1 -> MATLAB Function1/2(in1)
  Constant1/1 -> Sum1/1
  Sum1/1 -> Discrete-Time Integrator1/1  "x_dot"
  Discrete-Time Integrator/1 -> MATLAB Function1/1(in0)
  MATLAB Function1/1(out) -> Sum/2, MATLAB Function/1(x), Sum1/2  "x"
  low/1 -> MATLAB Function/3(LOW)
  high/1 -> MATLAB Function/4(HIGH)
  q/1 -> MATLAB Function1/3(ctrl), Discrete-Time Integrator1/2, Discrete-Time Integrator/2, MATLAB Function/2(q)

== system thermostat/Thermostat30 ==
  Constant : Constant  Value=10
  Constant1 : Constant  Value=37.78
  Discrete-Time Integrator : DiscreteIntegrator  ExternalReset=either  InitialCondition=25  InitialConditionSetting=State (most efficient)  SampleTime=-1
  Discrete-Time Integrator1 : DiscreteIntegrator  ExternalReset=either  InitialCondition=22.78  InitialConditionSetting=State (most efficient)  SampleTime=-1
  MATLAB Function : MATLAB Function  TreatAsAtomicUnit=on
  MATLAB Function1 : MATLAB Function  TreatAsAtomicUnit=on
  Sum : Sum  Inputs=|+-
  Sum1 : Sum  Inputs=|+-
  high : Constant  Value=25
  low : Constant  Value=22.78
  q : Memory
  wires:
  MATLAB Function/1(qNext) -> q/1
  Constant/1 -> Sum/1
  Sum/1 -> Discrete-Time Integrator/1  "x_dot"
  Discrete-Time Integrator1/1 -> MATLAB Function1/2(in1)
  Constant1/1 -> Sum1/1
  Sum1/1 -> Discrete-Time Integrator1/1  "x_dot"
  Discrete-Time Integrator/1 -> MATLAB Function1/1(in0)
  MATLAB Function1/1(out) -> Sum/2, MATLAB Function/1(x), Sum1/2  "x"
  low/1 -> MATLAB Function/3(LOW)
  high/1 -> MATLAB Function/4(HIGH)
  q/1 -> MATLAB Function1/3(ctrl), Discrete-Time Integrator1/2, Discrete-Time Integrator/2, MATLAB Function/2(q)

== system thermostat/Thermostat31 ==
  Constant : Constant  Value=10
  Constant1 : Constant  Value=37.78
  Discrete-Time Integrator : DiscreteIntegrator  ExternalReset=either  InitialCondition=25  InitialConditionSetting=State (most efficient)  SampleTime=-1
  Discrete-Time Integrator1 : DiscreteIntegrator  ExternalReset=either  InitialCondition=22.78  InitialConditionSetting=State (most efficient)  SampleTime=-1
  MATLAB Function : MATLAB Function  TreatAsAtomicUnit=on
  MATLAB Function1 : MATLAB Function  TreatAsAtomicUnit=on
  Sum : Sum  Inputs=|+-
  Sum1 : Sum  Inputs=|+-
  high : Constant  Value=25
  low : Constant  Value=22.78
  q : Memory
  wires:
  MATLAB Function/1(qNext) -> q/1
  Constant/1 -> Sum/1
  Sum/1 -> Discrete-Time Integrator/1  "x_dot"
  Discrete-Time Integrator1/1 -> MATLAB Function1/2(in1)
  Constant1/1 -> Sum1/1
  Sum1/1 -> Discrete-Time Integrator1/1  "x_dot"
  Discrete-Time Integrator/1 -> MATLAB Function1/1(in0)
  MATLAB Function1/1(out) -> Sum/2, MATLAB Function/1(x), Sum1/2  "x"
  low/1 -> MATLAB Function/3(LOW)
  high/1 -> MATLAB Function/4(HIGH)
  q/1 -> MATLAB Function1/3(ctrl), Discrete-Time Integrator1/2, Discrete-Time Integrator/2, MATLAB Function/2(q)

== system thermostat/Thermostat32 ==
  Constant : Constant  Value=10
  Constant1 : Constant  Value=37.78
  Discrete-Time Integrator : DiscreteIntegrator  ExternalReset=either  InitialCondition=25  InitialConditionSetting=State (most efficient)  SampleTime=-1
  Discrete-Time Integrator1 : DiscreteIntegrator  ExternalReset=either  InitialCondition=22.78  InitialConditionSetting=State (most efficient)  SampleTime=-1
  MATLAB Function : MATLAB Function  TreatAsAtomicUnit=on
  MATLAB Function1 : MATLAB Function  TreatAsAtomicUnit=on
  Sum : Sum  Inputs=|+-
  Sum1 : Sum  Inputs=|+-
  high : Constant  Value=25
  low : Constant  Value=22.78
  q : Memory
  wires:
  MATLAB Function/1(qNext) -> q/1
  Constant/1 -> Sum/1
  Sum/1 -> Discrete-Time Integrator/1  "x_dot"
  Discrete-Time Integrator1/1 -> MATLAB Function1/2(in1)
  Constant1/1 -> Sum1/1
  Sum1/1 -> Discrete-Time Integrator1/1  "x_dot"
  Discrete-Time Integrator/1 -> MATLAB Function1/1(in0)
  MATLAB Function1/1(out) -> Sum/2, MATLAB Function/1(x), Sum1/2  "x"
  low/1 -> MATLAB Function/3(LOW)
  high/1 -> MATLAB Function/4(HIGH)
  q/1 -> MATLAB Function1/3(ctrl), Discrete-Time Integrator1/2, Discrete-Time Integrator/2, MATLAB Function/2(q)

== system thermostat/Thermostat33 ==
  Constant : Constant  Value=10
  Constant1 : Constant  Value=37.78
  Discrete-Time Integrator : DiscreteIntegrator  ExternalReset=either  InitialCondition=25  InitialConditionSetting=State (most efficient)  SampleTime=-1
  Discrete-Time Integrator1 : DiscreteIntegrator  ExternalReset=either  InitialCondition=22.78  InitialConditionSetting=State (most efficient)  SampleTime=-1
  MATLAB Function : MATLAB Function  TreatAsAtomicUnit=on
  MATLAB Function1 : MATLAB Function  TreatAsAtomicUnit=on
  Sum : Sum  Inputs=|+-
  Sum1 : Sum  Inputs=|+-
  high : Constant  Value=25
  low : Constant  Value=22.78
  q : Memory
  wires:
  MATLAB Function/1(qNext) -> q/1
  Constant/1 -> Sum/1
  Sum/1 -> Discrete-Time Integrator/1  "x_dot"
  Discrete-Time Integrator1/1 -> MATLAB Function1/2(in1)
  Constant1/1 -> Sum1/1
  Sum1/1 -> Discrete-Time Integrator1/1  "x_dot"
  Discrete-Time Integrator/1 -> MATLAB Function1/1(in0)
  MATLAB Function1/1(out) -> Sum/2, MATLAB Function/1(x), Sum1/2  "x"
  low/1 -> MATLAB Function/3(LOW)
  high/1 -> MATLAB Function/4(HIGH)
  q/1 -> MATLAB Function1/3(ctrl), Discrete-Time Integrator1/2, Discrete-Time Integrator/2, MATLAB Function/2(q)

== system thermostat/Thermostat34 ==
  Constant : Constant  Value=10
  Constant1 : Constant  Value=37.78
  Discrete-Time Integrator : DiscreteIntegrator  ExternalReset=either  InitialCondition=25  InitialConditionSetting=State (most efficient)  SampleTime=-1
  Discrete-Time Integrator1 : DiscreteIntegrator  ExternalReset=either  InitialCondition=22.78  InitialConditionSetting=State (most efficient)  SampleTime=-1
  MATLAB Function : MATLAB Function  TreatAsAtomicUnit=on
  MATLAB Function1 : MATLAB Function  TreatAsAtomicUnit=on
  Sum : Sum  Inputs=|+-
  Sum1 : Sum  Inputs=|+-
  high : Constant  Value=25
  low : Constant  Value=22.78
  q : Memory
  wires:
  MATLAB Function/1(qNext) -> q/1
  Constant/1 -> Sum/1
  Sum/1 -> Discrete-Time Integrator/1  "x_dot"
  Discrete-Time Integrator1/1 -> MATLAB Function1/2(in1)
  Constant1/1 -> Sum1/1
  Sum1/1 -> Discrete-Time Integrator1/1  "x_dot"
  Discrete-Time Integrator/1 -> MATLAB Function1/1(in0)
  MATLAB Function1/1(out) -> Sum/2, MATLAB Function/1(x), Sum1/2  "x"
  low/1 -> MATLAB Function/3(LOW)
  high/1 -> MATLAB Function/4(HIGH)
  q/1 -> MATLAB Function1/3(ctrl), Discrete-Time Integrator1/2, Discrete-Time Integrator/2, MATLAB Function/2(q)

== system thermostat/Thermostat35 ==
  Constant : Constant  Value=10
  Constant1 : Constant  Value=37.78
  Discrete-Time Integrator : DiscreteIntegrator  ExternalReset=either  InitialCondition=25  InitialConditionSetting=State (most efficient)  SampleTime=-1
  Discrete-Time Integrator1 : DiscreteIntegrator  ExternalReset=either  InitialCondition=22.78  InitialConditionSetting=State (most efficient)  SampleTime=-1
  MATLAB Function : MATLAB Function  TreatAsAtomicUnit=on
  MATLAB Function1 : MATLAB Function  TreatAsAtomicUnit=on
  Sum : Sum  Inputs=|+-
  Sum1 : Sum  Inputs=|+-
  high : Constant  Value=25
  low : Constant  Value=22.78
  q : Memory
  wires:
  MATLAB Function/1(qNext) -> q/1
  Constant/1 -> Sum/1
  Sum/1 -> Discrete-Time Integrator/1  "x_dot"
  Discrete-Time Integrator1/1 -> MATLAB Function1/2(in1)
  Constant1/1 -> Sum1/1
  Sum1/1 -> Discrete-Time Integrator1/1  "x_dot"
  Discrete-Time Integrator/1 -> MATLAB Function1/1(in0)
  MATLAB Function1/1(out) -> Sum/2, MATLAB Function/1(x), Sum1/2  "x"
  low/1 -> MATLAB Function/3(LOW)
  high/1 -> MATLAB Function/4(HIGH)
  q/1 -> MATLAB Function1/3(ctrl), Discrete-Time Integrator1/2, Discrete-Time Integrator/2, MATLAB Function/2(q)

== system thermostat/Thermostat36 ==
  Constant : Constant  Value=10
  Constant1 : Constant  Value=37.78
  Discrete-Time Integrator : DiscreteIntegrator  ExternalReset=either  InitialCondition=25  InitialConditionSetting=State (most efficient)  SampleTime=-1
  Discrete-Time Integrator1 : DiscreteIntegrator  ExternalReset=either  InitialCondition=22.78  InitialConditionSetting=State (most efficient)  SampleTime=-1
  MATLAB Function : MATLAB Function  TreatAsAtomicUnit=on
  MATLAB Function1 : MATLAB Function  TreatAsAtomicUnit=on
  Sum : Sum  Inputs=|+-
  Sum1 : Sum  Inputs=|+-
  high : Constant  Value=25
  low : Constant  Value=22.78
  q : Memory
  wires:
  MATLAB Function/1(qNext) -> q/1
  Constant/1 -> Sum/1
  Sum/1 -> Discrete-Time Integrator/1  "x_dot"
  Discrete-Time Integrator1/1 -> MATLAB Function1/2(in1)
  Constant1/1 -> Sum1/1
  Sum1/1 -> Discrete-Time Integrator1/1  "x_dot"
  Discrete-Time Integrator/1 -> MATLAB Function1/1(in0)
  MATLAB Function1/1(out) -> Sum/2, MATLAB Function/1(x), Sum1/2  "x"
  low/1 -> MATLAB Function/3(LOW)
  high/1 -> MATLAB Function/4(HIGH)
  q/1 -> MATLAB Function1/3(ctrl), Discrete-Time Integrator1/2, Discrete-Time Integrator/2, MATLAB Function/2(q)

== system thermostat/Thermostat37 ==
  Constant : Constant  Value=10
  Constant1 : Constant  Value=37.78
  Discrete-Time Integrator : DiscreteIntegrator  ExternalReset=either  InitialCondition=25  InitialConditionSetting=State (most efficient)  SampleTime=-1
  Discrete-Time Integrator1 : DiscreteIntegrator  ExternalReset=either  InitialCondition=22.78  InitialConditionSetting=State (most efficient)  SampleTime=-1
  MATLAB Function : MATLAB Function  TreatAsAtomicUnit=on
  MATLAB Function1 : MATLAB Function  TreatAsAtomicUnit=on
  Sum : Sum  Inputs=|+-
  Sum1 : Sum  Inputs=|+-
  high : Constant  Value=25
  low : Constant  Value=22.78
  q : Memory
  wires:
  MATLAB Function/1(qNext) -> q/1
  Constant/1 -> Sum/1
  Sum/1 -> Discrete-Time Integrator/1  "x_dot"
  Discrete-Time Integrator1/1 -> MATLAB Function1/2(in1)
  Constant1/1 -> Sum1/1
  Sum1/1 -> Discrete-Time Integrator1/1  "x_dot"
  Discrete-Time Integrator/1 -> MATLAB Function1/1(in0)
  MATLAB Function1/1(out) -> Sum/2, MATLAB Function/1(x), Sum1/2  "x"
  low/1 -> MATLAB Function/3(LOW)
  high/1 -> MATLAB Function/4(HIGH)
  q/1 -> MATLAB Function1/3(ctrl), Discrete-Time Integrator1/2, Discrete-Time Integrator/2, MATLAB Function/2(q)

== system thermostat/Thermostat38 ==
  Constant : Constant  Value=10
  Constant1 : Constant  Value=37.78
  Discrete-Time Integrator : DiscreteIntegrator  ExternalReset=either  InitialCondition=25  InitialConditionSetting=State (most efficient)  SampleTime=-1
  Discrete-Time Integrator1 : DiscreteIntegrator  ExternalReset=either  InitialCondition=22.78  InitialConditionSetting=State (most efficient)  SampleTime=-1
  MATLAB Function : MATLAB Function  TreatAsAtomicUnit=on
  MATLAB Function1 : MATLAB Function  TreatAsAtomicUnit=on
  Sum : Sum  Inputs=|+-
  Sum1 : Sum  Inputs=|+-
  high : Constant  Value=25
  low : Constant  Value=22.78
  q : Memory
  wires:
  MATLAB Function/1(qNext) -> q/1
  Constant/1 -> Sum/1
  Sum/1 -> Discrete-Time Integrator/1  "x_dot"
  Discrete-Time Integrator1/1 -> MATLAB Function1/2(in1)
  Constant1/1 -> Sum1/1
  Sum1/1 -> Discrete-Time Integrator1/1  "x_dot"
  Discrete-Time Integrator/1 -> MATLAB Function1/1(in0)
  MATLAB Function1/1(out) -> Sum/2, MATLAB Function/1(x), Sum1/2  "x"
  low/1 -> MATLAB Function/3(LOW)
  high/1 -> MATLAB Function/4(HIGH)
  q/1 -> MATLAB Function1/3(ctrl), Discrete-Time Integrator1/2, Discrete-Time Integrator/2, MATLAB Function/2(q)

== system thermostat/Thermostat39 ==
  Constant : Constant  Value=10
  Constant1 : Constant  Value=37.78
  Discrete-Time Integrator : DiscreteIntegrator  ExternalReset=either  InitialCondition=25  InitialConditionSetting=State (most efficient)  SampleTime=-1
  Discrete-Time Integrator1 : DiscreteIntegrator  ExternalReset=either  InitialCondition=22.78  InitialConditionSetting=State (most efficient)  SampleTime=-1
  MATLAB Function : MATLAB Function  TreatAsAtomicUnit=on
  MATLAB Function1 : MATLAB Function  TreatAsAtomicUnit=on
  Sum : Sum  Inputs=|+-
  Sum1 : Sum  Inputs=|+-
  high : Constant  Value=25
  low : Constant  Value=22.78
  q : Memory
  wires:
  MATLAB Function/1(qNext) -> q/1
  Constant/1 -> Sum/1
  Sum/1 -> Discrete-Time Integrator/1  "x_dot"
  Discrete-Time Integrator1/1 -> MATLAB Function1/2(in1)
  Constant1/1 -> Sum1/1
  Sum1/1 -> Discrete-Time Integrator1/1  "x_dot"
  Discrete-Time Integrator/1 -> MATLAB Function1/1(in0)
  MATLAB Function1/1(out) -> Sum/2, MATLAB Function/1(x), Sum1/2  "x"
  low/1 -> MATLAB Function/3(LOW)
  high/1 -> MATLAB Function/4(HIGH)
  q/1 -> MATLAB Function1/3(ctrl), Discrete-Time Integrator1/2, Discrete-Time Integrator/2, MATLAB Function/2(q)

== system thermostat/Thermostat4 ==
  Constant : Constant  Value=10
  Constant1 : Constant  Value=37.78
  Discrete-Time Integrator : DiscreteIntegrator  ExternalReset=either  InitialCondition=25  InitialConditionSetting=State (most efficient)  SampleTime=-1
  Discrete-Time Integrator1 : DiscreteIntegrator  ExternalReset=either  InitialCondition=22.78  InitialConditionSetting=State (most efficient)  SampleTime=-1
  MATLAB Function : MATLAB Function  TreatAsAtomicUnit=on
  MATLAB Function1 : MATLAB Function  TreatAsAtomicUnit=on
  Sum : Sum  Inputs=|+-
  Sum1 : Sum  Inputs=|+-
  high : Constant  Value=25
  low : Constant  Value=22.78
  q : Memory
  wires:
  MATLAB Function/1(qNext) -> q/1
  Constant/1 -> Sum/1
  Sum/1 -> Discrete-Time Integrator/1  "x_dot"
  Discrete-Time Integrator1/1 -> MATLAB Function1/2(in1)
  Constant1/1 -> Sum1/1
  Sum1/1 -> Discrete-Time Integrator1/1  "x_dot"
  Discrete-Time Integrator/1 -> MATLAB Function1/1(in0)
  MATLAB Function1/1(out) -> Sum/2, MATLAB Function/1(x), Sum1/2  "x"
  low/1 -> MATLAB Function/3(LOW)
  high/1 -> MATLAB Function/4(HIGH)
  q/1 -> MATLAB Function1/3(ctrl), Discrete-Time Integrator1/2, Discrete-Time Integrator/2, MATLAB Function/2(q)

== system thermostat/Thermostat40 ==
  Constant : Constant  Value=10
  Constant1 : Constant  Value=37.78
  Discrete-Time Integrator : DiscreteIntegrator  ExternalReset=either  InitialCondition=25  InitialConditionSetting=State (most efficient)  SampleTime=-1
  Discrete-Time Integrator1 : DiscreteIntegrator  ExternalReset=either  InitialCondition=22.78  InitialConditionSetting=State (most efficient)  SampleTime=-1
  MATLAB Function : MATLAB Function  TreatAsAtomicUnit=on
  MATLAB Function1 : MATLAB Function  TreatAsAtomicUnit=on
  Sum : Sum  Inputs=|+-
  Sum1 : Sum  Inputs=|+-
  high : Constant  Value=25
  low : Constant  Value=22.78
  q : Memory
  wires:
  MATLAB Function/1(qNext) -> q/1
  Constant/1 -> Sum/1
  Sum/1 -> Discrete-Time Integrator/1  "x_dot"
  Discrete-Time Integrator1/1 -> MATLAB Function1/2(in1)
  Constant1/1 -> Sum1/1
  Sum1/1 -> Discrete-Time Integrator1/1  "x_dot"
  Discrete-Time Integrator/1 -> MATLAB Function1/1(in0)
  MATLAB Function1/1(out) -> Sum/2, MATLAB Function/1(x), Sum1/2  "x"
  low/1 -> MATLAB Function/3(LOW)
  high/1 -> MATLAB Function/4(HIGH)
  q/1 -> MATLAB Function1/3(ctrl), Discrete-Time Integrator1/2, Discrete-Time Integrator/2, MATLAB Function/2(q)

== system thermostat/Thermostat41 ==
  Constant : Constant  Value=10
  Constant1 : Constant  Value=37.78
  Discrete-Time Integrator : DiscreteIntegrator  ExternalReset=either  InitialCondition=25  InitialConditionSetting=State (most efficient)  SampleTime=-1
  Discrete-Time Integrator1 : DiscreteIntegrator  ExternalReset=either  InitialCondition=22.78  InitialConditionSetting=State (most efficient)  SampleTime=-1
  MATLAB Function : MATLAB Function  TreatAsAtomicUnit=on
  MATLAB Function1 : MATLAB Function  TreatAsAtomicUnit=on
  Sum : Sum  Inputs=|+-
  Sum1 : Sum  Inputs=|+-
  high : Constant  Value=25
  low : Constant  Value=22.78
  q : Memory
  wires:
  MATLAB Function/1(qNext) -> q/1
  Constant/1 -> Sum/1
  Sum/1 -> Discrete-Time Integrator/1  "x_dot"
  Discrete-Time Integrator1/1 -> MATLAB Function1/2(in1)
  Constant1/1 -> Sum1/1
  Sum1/1 -> Discrete-Time Integrator1/1  "x_dot"
  Discrete-Time Integrator/1 -> MATLAB Function1/1(in0)
  MATLAB Function1/1(out) -> Sum/2, MATLAB Function/1(x), Sum1/2  "x"
  low/1 -> MATLAB Function/3(LOW)
  high/1 -> MATLAB Function/4(HIGH)
  q/1 -> MATLAB Function1/3(ctrl), Discrete-Time Integrator1/2, Discrete-Time Integrator/2, MATLAB Function/2(q)

== system thermostat/Thermostat42 ==
  Constant : Constant  Value=10
  Constant1 : Constant  Value=37.78
  Discrete-Time Integrator : DiscreteIntegrator  ExternalReset=either  InitialCondition=25  InitialConditionSetting=State (most efficient)  SampleTime=-1
  Discrete-Time Integrator1 : DiscreteIntegrator  ExternalReset=either  InitialCondition=22.78  InitialConditionSetting=State (most efficient)  SampleTime=-1
  MATLAB Function : MATLAB Function  TreatAsAtomicUnit=on
  MATLAB Function1 : MATLAB Function  TreatAsAtomicUnit=on
  Sum : Sum  Inputs=|+-
  Sum1 : Sum  Inputs=|+-
  high : Constant  Value=25
  low : Constant  Value=22.78
  q : Memory
  wires:
  MATLAB Function/1(qNext) -> q/1
  Constant/1 -> Sum/1
  Sum/1 -> Discrete-Time Integrator/1  "x_dot"
  Discrete-Time Integrator1/1 -> MATLAB Function1/2(in1)
  Constant1/1 -> Sum1/1
  Sum1/1 -> Discrete-Time Integrator1/1  "x_dot"
  Discrete-Time Integrator/1 -> MATLAB Function1/1(in0)
  MATLAB Function1/1(out) -> Sum/2, MATLAB Function/1(x), Sum1/2  "x"
  low/1 -> MATLAB Function/3(LOW)
  high/1 -> MATLAB Function/4(HIGH)
  q/1 -> MATLAB Function1/3(ctrl), Discrete-Time Integrator1/2, Discrete-Time Integrator/2, MATLAB Function/2(q)

== system thermostat/Thermostat43 ==
  Constant : Constant  Value=10
  Constant1 : Constant  Value=37.78
  Discrete-Time Integrator : DiscreteIntegrator  ExternalReset=either  InitialCondition=25  InitialConditionSetting=State (most efficient)  SampleTime=-1
  Discrete-Time Integrator1 : DiscreteIntegrator  ExternalReset=either  InitialCondition=22.78  InitialConditionSetting=State (most efficient)  SampleTime=-1
  MATLAB Function : MATLAB Function  TreatAsAtomicUnit=on
  MATLAB Function1 : MATLAB Function  TreatAsAtomicUnit=on
  Sum : Sum  Inputs=|+-
  Sum1 : Sum  Inputs=|+-
  high : Constant  Value=25
  low : Constant  Value=22.78
  q : Memory
  wires:
  MATLAB Function/1(qNext) -> q/1
  Constant/1 -> Sum/1
  Sum/1 -> Discrete-Time Integrator/1  "x_dot"
  Discrete-Time Integrator1/1 -> MATLAB Function1/2(in1)
  Constant1/1 -> Sum1/1
  Sum1/1 -> Discrete-Time Integrator1/1  "x_dot"
  Discrete-Time Integrator/1 -> MATLAB Function1/1(in0)
  MATLAB Function1/1(out) -> Sum/2, MATLAB Function/1(x), Sum1/2  "x"
  low/1 -> MATLAB Function/3(LOW)
  high/1 -> MATLAB Function/4(HIGH)
  q/1 -> MATLAB Function1/3(ctrl), Discrete-Time Integrator1/2, Discrete-Time Integrator/2, MATLAB Function/2(q)
